simulink model "cav_mpc"  (R2026b)
settings: Solver=ode4  StopTime=P.Tsim  FixedStep=P.dt
InitFcn:
  | P = cav_params(); road = make_road(P.road.segments, P.road.ds, P.road.transition); mpcverbosity off;
libraries: mpcadaslib x2, autolibshared x1
settings Model: Creator=za  LastModifiedBy=za
settings SolverCC: AutoInsertRateTranBlk=on

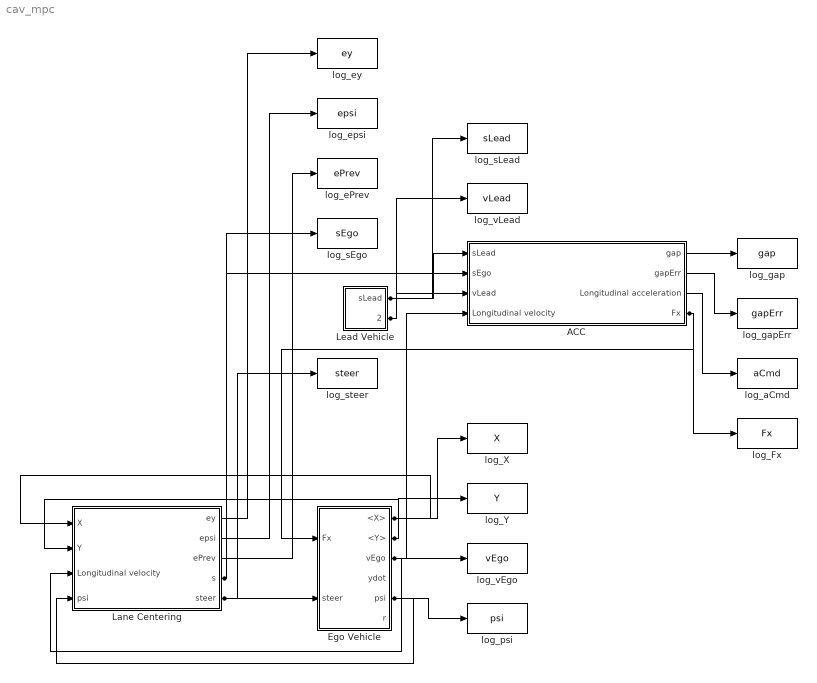
== system cav_mpc ==
  ACC : Subsystem
  Ego Vehicle : Subsystem
  Lane Centering : Subsystem
  Lead Vehicle : Subsystem
  log_Fx : ToWorkspace  VariableName=Fx  SaveFormat=Timeseries  SampleTime=P.Ts
  log_X : ToWorkspace  VariableName=X  SaveFormat=Timeseries  SampleTime=P.Ts
  log_Y : ToWorkspace  VariableName=Y  SaveFormat=Timeseries  SampleTime=P.Ts
  log_aCmd : ToWorkspace  VariableName=aCmd  SaveFormat=Timeseries  SampleTime=P.Ts
  log_ePrev : ToWorkspace  VariableName=ePrev  SaveFormat=Timeseries  SampleTime=P.Ts
  log_epsi : ToWorkspace  VariableName=epsi  SaveFormat=Timeseries  SampleTime=P.Ts
  log_ey : ToWorkspace  VariableName=ey  SaveFormat=Timeseries  SampleTime=P.Ts
  log_gap : ToWorkspace  VariableName=gap  SaveFormat=Timeseries  SampleTime=P.Ts
  log_gapErr : ToWorkspace  VariableName=gapErr  SaveFormat=Timeseries  SampleTime=P.Ts
  log_psi : ToWorkspace  VariableName=psi  SaveFormat=Timeseries  SampleTime=P.Ts
  log_sEgo : ToWorkspace  VariableName=sEgo  SaveFormat=Timeseries  SampleTime=P.Ts
  log_sLead : ToWorkspace  VariableName=sLead  SaveFormat=Timeseries  SampleTime=P.Ts
  log_steer : ToWorkspace  VariableName=steer  SaveFormat=Timeseries  SampleTime=P.Ts
  log_vEgo : ToWorkspace  VariableName=vEgo  SaveFormat=Timeseries  SampleTime=P.Ts
  log_vLead : ToWorkspace  VariableName=vLead  SaveFormat=Timeseries  SampleTime=P.Ts
  wires:
  ACC/3(Longitudinal acceleration) -> log_aCmd/1
  ACC/4(Fx) -> log_Fx/1, Ego Vehicle/1(Fx)
  Lane Centering/1(ey) -> log_ey/1
  Lane Centering/3(ePrev) -> log_ePrev/1
  Lane Centering/5(steer) -> Ego Vehicle/2(steer), log_steer/1
  Lane Centering/2(epsi) -> log_epsi/1
  Lane Centering/4(s) -> log_sEgo/1, ACC/2(sEgo)
  ACC/1(gap) -> log_gap/1
  Lead Vehicle/1(sLead) -> ACC/1(sLead), log_sLead/1
  Lead Vehicle/2(vLead) -> log_vLead/1, ACC/3(vLead)
  Ego Vehicle/1(<X>) -> log_X/1, Lane Centering/1(X)
  Ego Vehicle/3(vEgo) -> ACC/4(Longitudinal velocity), log_vEgo/1, Lane Centering/3(Longitudinal velocity)
  Ego Vehicle/2(<Y>) -> log_Y/1, Lane Centering/2(Y)
  Ego Vehicle/5(psi) -> log_psi/1, Lane Centering/4(psi)
  ACC/2(gapErr) -> log_gapErr/1

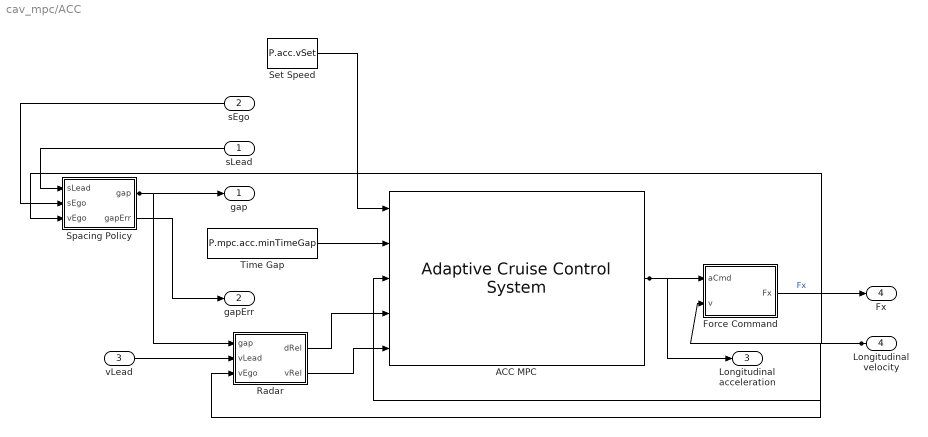
== system cav_mpc/ACC ==
  sLead : Inport
  sEgo : Inport  Port=2
  vLead : Inport  Port=3
  Longitudinal velocity : Inport  Port=4
  ACC MPC : mpcadaslib/Adaptive Cruise Control System  EgoModel=tf(1, [0.15 1 0])  InitialEgoVelocity=20  DefaultSpacing=6  MaxVelocity=50  MinAcceleration=-4  amin_ext=off  MaxAcceleration=2  amax_ext=off  Ts=0.1  PredictionHorizon=30  ControllerBehavior=0.5  suboptimal=off  maxiter=10  datatypeopt=double  optmode=off  trackmode=off
      settings: LibrarySourceBlock=mpclib/Automated Driving/Adaptive Cruise Control System
  Force Command : MATLAB Function  TreatAsAtomicUnit=on
  Radar : MATLAB Function  TreatAsAtomicUnit=on
  Set Speed : Constant  Value=P.acc.vSet
  Spacing Policy : MATLAB Function  TreatAsAtomicUnit=on
  Time Gap : Constant  Value=P.mpc.acc.minTimeGap
  gap : Outport
  gapErr : Outport  Port=2
  Longitudinal acceleration : Outport  Port=3
  Fx : Outport  Port=4
  wires:
  Longitudinal velocity/1 -> ACC MPC/3, Force Command/2(v), Radar/3(vEgo), Spacing Policy/3(vEgo)
  Radar/1(dRel) -> ACC MPC/4
  Force Command/1(Fx) -> Fx/1  "Fx"
  Time Gap/1 -> ACC MPC/2
  Set Speed/1 -> ACC MPC/1
  sLead/1 -> Spacing Policy/1(sLead)
  Radar/2(vRel) -> ACC MPC/5
  sEgo/1 -> Spacing Policy/2(sEgo)
  Spacing Policy/2(gapErr) -> gapErr/1
  ACC MPC/1 -> Longitudinal acceleration/1, Force Command/1(aCmd)
  vLead/1 -> Radar/2(vLead)
  Spacing Policy/1(gap) -> gap/1, Radar/1(gap)

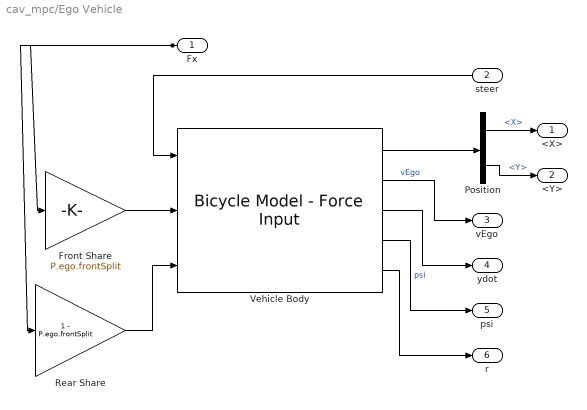
== system cav_mpc/Ego Vehicle ==
  Fx : Inport
  steer : Inport  Port=2
  Front Share : Gain  Gain=P.ego.frontSplit
  Position : BusSelector  OutputSignals=InertFrm.Cg.Disp.X,InertFrm.Cg.Disp.Y
  Rear Share : Gain  Gain=1 - P.ego.frontSplit
  Vehicle Body : autolibshared/Bicycle Model - Force Input  trackMode=Single (bicycle)  inputMode=External longitudinal forces  frontSteerMode=on  rearSteerMode=off  windMode=off  muMode=off  extFMode=off  extMMode=off  aMode=2  NF=2  NR=2  m=P.ego.m  a=P.ego.a  b=P.ego.b  h=0.35  X_o=0  xdot_o=P.ego.v0  CalphaMode=Constant  sigmaMode=on  w=[1.4,1.4]  Cy_f=P.ego.Cyf  Cy_r=P.ego.Cyr  sigma_f=.1  sigma_r=.1  alpha_f_brk=[-.1 .1]  Cy_f_data=[-9e3 9e3]  alpha_r_brk=[-.1 .1]  Cy_r_data=[-9e3 9e3]  Y_o=0  ydot_o=0  Izz=P.ego.Izz  psi_o=0  r_o=0  Af=2  Cd=.3  Cl=.1  Cpm=.1  beta_w=[0,0.1745,0.3491,0.5236,0.6981,0.8727,1.0472,1.2217,1.3963,1.5708]  Cs=[0.1000,0.1000,0.1000,0.1000,0.1000,0.1000,0.1000,0.1000,0.1000,0.1000]  Cym=[0,0,0.0667,0.1000,0.1333,0.1667,0.2000,0.2333,0.2667,0.3000]  Pabs=101325  Tair=273  g=9.81  mu=1  xdot_tol=0.1  Fznom=5000  Fxtire_sat=1e6  Fytire_sat=1e6  longOff=0  latOff=0  vertOff=0.35
      settings: LibrarySourceBlock=vehdynlibeom/Bicycle Model - Force Input
  <X> : Outport
  <Y> : Outport  Port=2
  vEgo : Outport  Port=3
  ydot : Outport  Port=4
  psi : Outport  Port=5
  r : Outport  Port=6
  wires:
  Position/2 -> <Y>/1  "<Y>"
  Vehicle Body/4 -> psi/1  "psi"
  Vehicle Body/5 -> r/1
  Vehicle Body/3 -> ydot/1
  Vehicle Body/2 -> vEgo/1  "vEgo"
  Vehicle Body/1 -> Position/1
  Position/1 -> <X>/1  "<X>"
  Fx/1 -> Rear Share/1, Front Share/1
  steer/1 -> Vehicle Body/1
  Rear Share/1 -> Vehicle Body/3
  Front Share/1 -> Vehicle Body/2

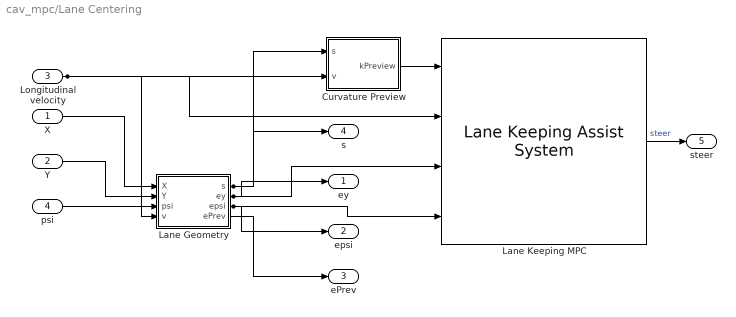
== system cav_mpc/Lane Centering ==
  X : Inport
  Y : Inport  Port=2
  Longitudinal velocity : Inport  Port=3
  psi : Inport  Port=4
  Curvature Preview : MATLAB Function  TreatAsAtomicUnit=on
  Lane Geometry : MATLAB Function  TreatAsAtomicUnit=on
  Lane Keeping MPC : mpcadaslib/Lane Keeping Assist System  ModelType=Use vehicle parameters  VehicleMass=2000  VehicleYawInertia=4000  LengthToFront=1.4  LengthToRear=1.6  FrontTireStiffness=80000  RearTireStiffness=75000  EgoModelMatrixA=[-4.4021 ,-12.4603;1.3913,-5.1868]  EgoModelMatrixB=[24.1270;15.8609]  EgoModelMatrixC=[1,0;0,1]  InitialLongVel=20  TransportLag=0  MinSteering=-0.523599  umin_ext=off  MaxSteering=0.523599  umax_ext=off  Ts=0.1  PredictionHorizon=20  ControllerBehavior=0.5  suboptimal=off  maxiter=10  datatypeopt=double  optmode=off  trackmode=off
      settings: LibrarySourceBlock=mpclib/Automated Driving/Lane Keeping Assist System
  ey : Outport
  epsi : Outport  Port=2
  ePrev : Outport  Port=3
  s : Outport  Port=4
  steer : Outport  Port=5
  wires:
  Lane Keeping MPC/1 -> steer/1  "steer"
  Curvature Preview/1(kPreview) -> Lane Keeping MPC/1
  Lane Geometry/4(ePrev) -> ePrev/1
  Lane Geometry/3(epsi) -> epsi/1, Lane Keeping MPC/4
  Lane Geometry/2(ey) -> ey/1, Lane Keeping MPC/3
  Lane Geometry/1(s) -> Curvature Preview/1(s), s/1
  psi/1 -> Lane Geometry/3(psi)
  Y/1 -> Lane Geometry/2(Y)
  X/1 -> Lane Geometry/1(X)
  Longitudinal velocity/1 -> Lane Geometry/4(v), Lane Keeping MPC/2, Curvature Preview/2(v)

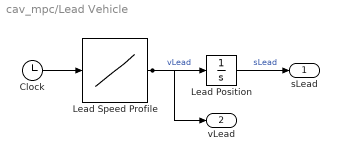
== system cav_mpc/Lead Vehicle ==
  Clock : Clock
  Lead Position : Integrator  InitialCondition=P.lead.s0
  Lead Speed Profile : Lookup_n-D  NumberOfTableDimensions=1  BreakpointsForDimension1=P.lead.t  Table=P.lead.v  ExtrapMethod=Clip  InternalRulePriority=Speed  RndMeth=Simplest
  sLead : Outport
  vLead : Outport  Port=2
  wires:
  Lead Position/1 -> sLead/1  "sLead"
  Lead Speed Profile/1 -> Lead Position/1, vLead/1  "vLead"
  Clock/1 -> Lead Speed Profile/1

== matlab function cav_mpc/ACC/Spacing Policy ==
  settings: updateMethod=DISCRETE  sampleTime=P.Ts
  data: sLead input; gap output; sEgo input; vEgo input; gapErr output; P parameter
function [gap, gapErr] = spacing_policy(sLead, sEgo, vEgo, P)
%Bumper-to-bumper gap and its error from the constant time-gap policy.
gap = sLead - sEgo - (P.ego.length + P.lead.length) / 2;
gapErr = gap - (P.acc.d0 + P.acc.Th * vEgo);
end

== matlab function cav_mpc/Lane Centering/Lane Geometry ==
  settings: updateMethod=DISCRETE  sampleTime=P.Ts
  data: X input; s output; Y input; psi input; v input; ey output; epsi output; ePrev output; road parameter; P parameter
function [s, ey, epsi, ePrev] = lane_geometry(X, Y, psi, v, road, P)
%Arc length, lateral offset (left positive), heading error, and the
%lookahead error the steering PID drives to 0: the offset of a point L
%ahead along the heading, measured from the lane tangent at the car. It
%is zero only when the car is centered and aligned, so on a curve the
%integral term supplies the steady steering.
persistent idx
n = numel(road.x);
if isempty(idx)
    idx = nearest_index(road, X, Y, 1, n);
else
    idx = nearest_index(road, X, Y, max(1, idx - 40), min(n, idx + 200));
end
%Interpolate along the arc between centerline points, so heading and
%offset change smoothly instead of in steps of ds * curvature.
dx = X - road.x(idx);
dy = Y - road.y(idx);
along = cos(road.th(idx)) * dx + sin(road.th(idx)) * dy;
th = road.th(idx) + road.k(idx) * along;
ey = -sin(road.th(idx)) * dx + cos(road.th(idx)) * dy - road.k(idx) * along^2 / 2;
s = road.s(idx) + along;
epsi = atan2(sin(psi - th), cos(psi - th));
L = P.lat.L0 + P.lat.Tla * max(v, 0);
ePrev = ey + L * sin(epsi);
end

function best = nearest_index(road, X, Y, lo, hi)
best = lo;
bestD = inf;
for k = lo:hi
    d = (road.x(k) - X)^2 + (road.y(k) - Y)^2;
    if d < bestD
        bestD = d;
        best = k;
    end
end
end

== matlab function cav_mpc/Lane Centering/Curvature Preview ==
  settings: updateMethod=DISCRETE  sampleTime=P.mpc.Ts
  data: s input; kPreview output; v input; road parameter; P parameter
function kPreview = curvature_preview(s, v, road, P)
%Road curvature at each step of the MPC prediction horizon, assuming the
%car holds its current speed.
p = P.mpc.lat.horizon;
kPreview = zeros(1, p);
n = numel(road.k);
for j = 1:p
    i = round((s + max(v, 0) * P.mpc.Ts * j) / road.ds) + 1;
    kPreview(j) = road.k(min(max(i, 1), n));
end
end

== matlab function cav_mpc/ACC/Radar ==
  settings: updateMethod=DISCRETE  sampleTime=P.Ts
  data: gap input; dRel output; vLead input; vEgo input; vRel output; P parameter
function [dRel, vRel] = radar(gap, vLead, vEgo, P)
%Relative distance and speed of the lead, or a clear road beyond range.
if gap < P.acc.range
    dRel = gap;
    vRel = vLead - vEgo;
else
    dRel = 1000;
    vRel = 0;
end
end

== matlab function cav_mpc/ACC/Force Command ==
  settings: updateMethod=DISCRETE  sampleTime=P.Ts
  data: aCmd input; Fx output; v input; P parameter
function Fx = force_command(aCmd, v, P)
%Axle force for the commanded acceleration, plus aerodynamic drag.
Fx = P.ego.m * aCmd + P.ego.cDrag * v^2;
Fx = min(max(Fx, P.acc.FxMin), P.acc.FxMax);
end
